simulink model "msk_sys"  (R2019b)
settings: Solver=VariableStepAuto  StartTime=0.0  StopTime=0.1  RelTol=1e-3
libraries: commdigbbndfm2 x2, commchan3 x1, commrandsrc3 x1, commsink2 x1
settings Model: Creator=yango  LastModifiedBy=yango

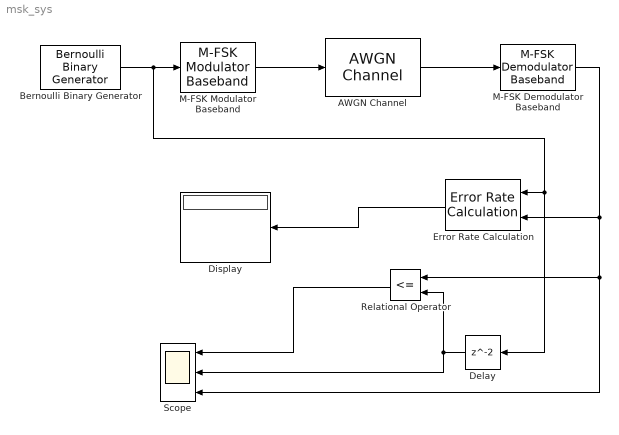
== system msk_sys ==
  AWGN Channel : commchan3/AWGN Channel  InputProcessing=Columns as channels (frame based)  seed=67  noiseMode="Signal to noise ratio  (Eb/No)"  EbNodB=12  EsNodB=10  SNRdB=10  bitsPerSym=1  Ps=1  Tsym=1/1200  variance=1
      settings: SourceProductName=Communications Toolbox
  Bernoulli Binary Generator : commrandsrc3/Bernoulli Binary Generator  ProbabilityOfZero=0.5  SeedSource=Auto  Seed=0  SampleTime=1/1200  SamplesPerFrame=1  OutputDataType=double  SimulateUsing=Interpreted execution
      settings: SourceProductName=Communications Toolbox
  Delay : Delay
  Display : Display
  Error Rate Calculation : commsink2/Error Rate Calculation  N=0  st_delay=0  cp_mode=Entire frame  subframe=[]  PMode=Port  WsName=ErrorVec  RsMode2=off  stop=off  numErr=100  maxBits=1e6
      settings: SourceProductName=Communications Toolbox
  M-FSK Demodulator Baseband : commdigbbndfm2/M-FSK Demodulator Baseband  M=2  OutType=Integer  Dec=Gray  freqSep=1000  numSamp=1200  RateOptions=Enforce single-rate processing  outDataType=double
      settings: SourceProductName=Communications Toolbox  SourceProductBaseCode=CM
  M-FSK Modulator Baseband : commdigbbndfm2/M-FSK Modulator Baseband  M=2  InType=Integer  Enc=Gray  freqSep=1000  phaseType=Continuous  numSamp=1200  RateOptions=Enforce single-rate processing  outDataType=double
      settings: SourceProductName=Communications Toolbox
  Relational Operator : RelationalOperator  Operator=<=  OutDataTypeStr=boolean  RndMeth=Simplest
  Scope : Scope  NumInputPorts=3
  wires:
  Bernoulli Binary Generator/1 -> Delay/1, Error Rate Calculation/1, M-FSK Modulator Baseband/1
  M-FSK Modulator Baseband/1 -> AWGN Channel/1
  AWGN Channel/1 -> M-FSK Demodulator Baseband/1
  Error Rate Calculation/1 -> Display/1
  M-FSK Demodulator Baseband/1 -> Relational Operator/1, Scope/3, Error Rate Calculation/2
  Delay/1 -> Relational Operator/2, Scope/2
  Relational Operator/1 -> Scope/1
